simulink model "CBE_145_HW4_P2a"  (R2021b)
settings: Solver=VariableStepAuto  StartTime=0.0  StopTime=25  RelTol=1e-3
settings Model: SimulationMode=rapid-accelerator  Creator=Jesus Vergara  LastModifiedBy=brame
settings SolverCC: AlgebraicLoopSolver=TrustRegion
settings DebuggingCC: SFMachineParentedDataDiag=warning

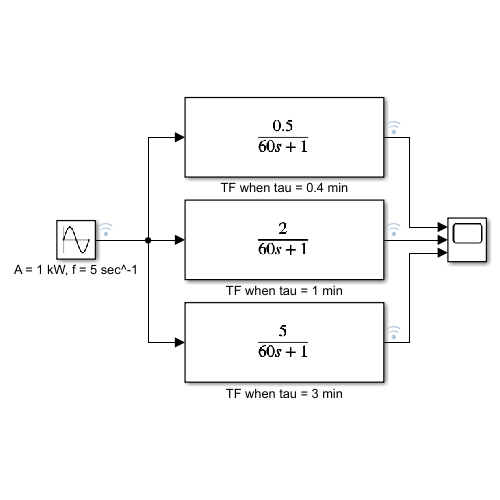
[thumbnail: Simulink's stored preview of the top-level diagram]
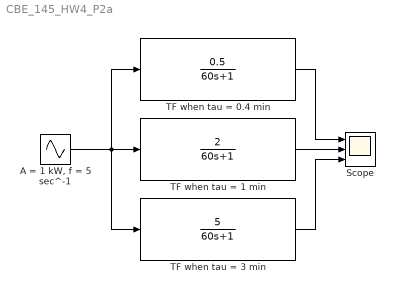
== system CBE_145_HW4_P2a ==
  "A = 1 kW, f = 5 sec^-1" : Sin  Frequency=5  SampleTime=0
  Scope : Scope  NumInputPorts=3
  TF when tau = 0.4 min : TransferFcn  Numerator=[0.5]  Denominator=[60 1]
  TF when tau = 1 min : TransferFcn  Numerator=[2]  Denominator=[60 1]
  TF when tau = 3 min : TransferFcn  Numerator=[5]  Denominator=[60 1]
  wires:
  "A = 1 kW, f = 5 sec^-1"/1 -> TF when tau = 3 min/1, TF when tau = 0.4 min/1, TF when tau = 1 min/1
  TF when tau = 1 min/1 -> Scope/2
  TF when tau = 0.4 min/1 -> Scope/1
  TF when tau = 3 min/1 -> Scope/3
